simulink model "malha_aberta"  (R2023a)
settings: Solver=VariableStepAuto  StartTime=0.0  StopTime=sampletime  RelTol=1e-3
undefined symbols (not defined in the file or in its folder): A, Gn, Is, Iscn, K1, L, Rp, Rs, Tn, Vi
settings Model: Creator=05630646761  LastModifiedBy=pedro
settings SolverCC: AlgebraicLoopSolver=TrustRegion
settings DataIOCC: ReturnWorkspaceOutputs=off
settings DebuggingCC: UnconnectedInputMsg=warning  UnconnectedOutputMsg=warning  UnconnectedLineMsg=warning  ArithmeticOperatorsInVariantConditions=warning
settings ModelReferenceCC: EnableRefExpFcnMdlSchedulingChecks=on
settings SFSimCC: SimUseLocalCustomCode=off  CustomCodeUndefinedFunction=UseInterfaceOnly
settings RTWCC: RTWUseLocalCustomCode=off
settings CodeAppCC: StateflowObjectComments=on

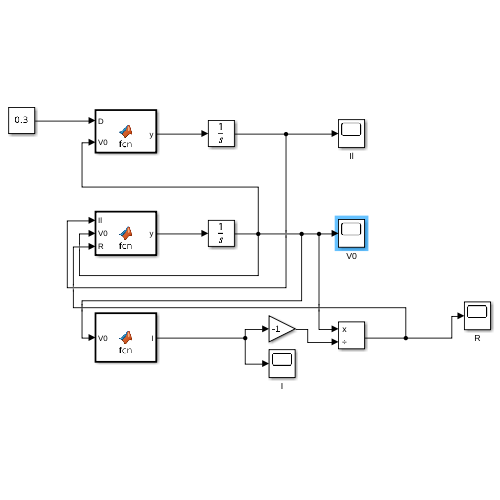
[thumbnail: Simulink's stored preview of the top-level diagram]
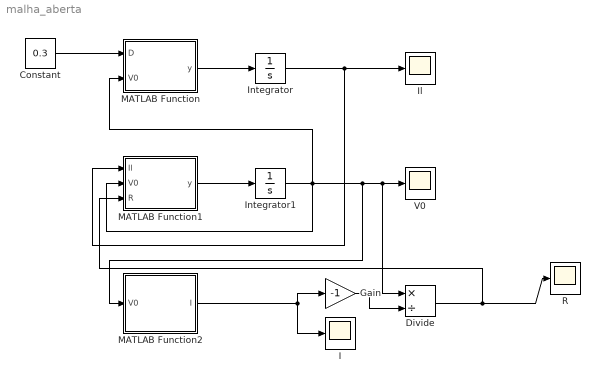
== system malha_aberta ==
  Constant : Constant  Value=0.3
  Divide : Product  Inputs=*/
  Gain : Gain  Gain=-1
  I : Scope
  Il : Scope
  Integrator : Integrator
  Integrator1 : Integrator  InitialCondition=0.6
  MATLAB Function : MATLAB Function  TreatAsAtomicUnit=on
  MATLAB Function1 : MATLAB Function  TreatAsAtomicUnit=on
  MATLAB Function2 : MATLAB Function  TreatAsAtomicUnit=on
  R : Scope
  V0 : Scope
  wires:
  MATLAB Function/1(y) -> Integrator/1
  MATLAB Function1/1(y) -> Integrator1/1
  Constant/1 -> MATLAB Function/1(D)
  MATLAB Function2/1(I) -> Gain/1, I/1
  Integrator/1 -> Il/1, MATLAB Function1/1(Il)
  Integrator1/1 -> MATLAB Function2/1(V0), Divide/1, V0/1, MATLAB Function1/2(V0), MATLAB Function/2(V0)
  Divide/1 -> MATLAB Function1/3(R), R/1
  Gain/1 -> Divide/2

== matlab function malha_aberta/MATLAB Function1 ==
  data: Il input; y output; V0 input; C parameter; R input
function y = fcn(Il, V0, C, R)

    y = (Il/C) - (V0/(R*C));

== matlab function malha_aberta/MATLAB Function ==
  data: D input; y output; V0 input; L parameter; Vi parameter
function y = fcn(D, V0, L, Vi)

    y = (D*Vi/L) - V0/L;

== matlab function malha_aberta/MATLAB Function2 ==
  data: V0 input; I output; Gn parameter; Iscn parameter; K1 parameter; Tn parameter; Is parameter; Rs parameter; A parameter; Rp parameter
function I = fcn(V0, Gn, Iscn, K1, Tn, Is, Rs, A, Rp)

G = Gn;
lambida = 0.1;
q = 1.602*(10^(-19)); %[C]
k = 1.38 *(10^(-23));
tol = 0.005;
 
%%
 
T = 0+273; 
Init = 0.5;     
Vt = k*T/q;
Inov = Init;
var = tol*2;
    
  while abs(var) > tol
          Iant = Inov;
          Ipv = (G/Gn)*(Iscn + K1*(T-Tn));
          Id = Is*(exp((V0 + Rs*Iant)/(Vt*A)) - 1);
          Ip = ((V0 + Rs*Iant)/Rp);
          Inov = Ipv - Id - Ip;
          Inov = lambida*Inov + (1 - lambida)*Iant;
          var = Inov - Iant;
   end    
       I = Inov;
